simulink model "Ex3_3"  (R2019b)
settings: Solver=VariableStepAuto  StartTime=0.0  StopTime=inf  RelTol=1e-3
values from neighbouring files (symbols this model uses):
  attMtx = [L*k, 0, -L*k, 0; 0, L*k, 0, -L*k; b, -b, b, -b; 1, 1, 1, 1]    [Ex6_3_constants.m]
  b = 1.3678e-07    [Ex6_3_constants.m]
  D = diag([kD, kD, kD])    [Ex6_3_constants.m]
  g = [0, 0, -9.81]'    [Ex6_3_constants.m]
  I = diag([Ixx, Iyy, Izz])    [Ex6_3_constants.m]
  Ixx = 0.007    [Ex6_3_constants.m]
  Iyy = 0.007    [Ex6_3_constants.m]
  Izz = 0.012    [Ex6_3_constants.m]
  k = 8.54858e-06    [Ex6_3_constants.m]
  L = 0.17    [Ex6_3_constants.m]
  m = 0.716    [Ex6_3_constants.m]
  mmat = diag([m, m, m])    [Ex6_3_constants.m]
  posMtx = [0, -1, 0; 1, 0, 0]    [Ex6_3_constants.m]
undefined symbols (not defined in the file or in its folder): AA, BB, CC, DD, Omega
libraries: simulink x6, vrlib x1
settings Model: Creator=ubuntu  LastModifiedBy=ubuntu

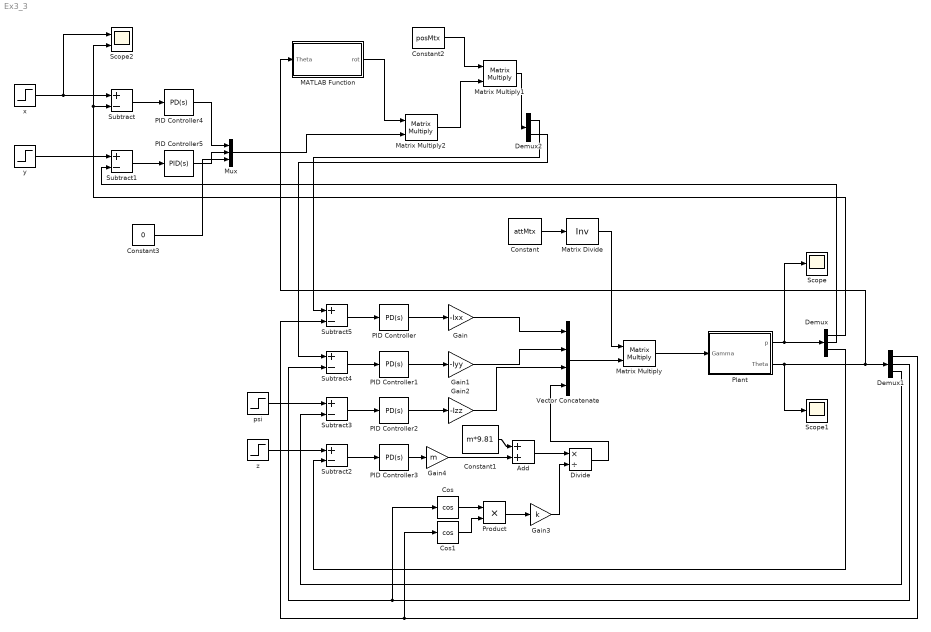
== system Ex3_3 ==
  Add : Sum
  Constant : Constant  Value=attMtx
  Constant1 : Constant  Value=m*9.81
  Constant2 : Constant  Value=posMtx
  Constant3 : Constant  Value=0
  Cos : Trigonometry  Operator=cos
  Cos1 : Trigonometry  Operator=cos
  Demux : Demux  Outputs=3
  Demux1 : Demux  Outputs=3
  Demux2 : Demux  Outputs=2
  Divide : Product  Inputs=*/
  Gain : Gain  Gain=-Ixx
  Gain1 : Gain  Gain=-Iyy
  Gain2 : Gain  Gain=-Izz
  Gain3 : Gain  Gain=k
  Gain4 : Gain  Gain=m
  MATLAB Function : MATLAB Function  TreatAsAtomicUnit=on
  Matrix Divide : Product  Inputs=/  Multiplication=Matrix(*)
  Matrix Multiply : Product  Multiplication=Matrix(*)
  Matrix Multiply1 : Product  Multiplication=Matrix(*)
  Matrix Multiply2 : Product  Multiplication=Matrix(*)
  Mux : Mux  Inputs=3
  PID Controller : simulink/Continuous/PID Controller  Controller=PD  Form=Parallel  TimeDomain=Continuous-time  SampleTime=-1  IntegratorMethod=Forward Euler  FilterMethod=Forward Euler  ControllerParametersSource=internal  P=-0.0546888957134836  I=1  D=-2.49980858398748  UseFilter=on  N=285.7069940104  TunerSelectOption=Transfer Function Based (PID Tuner App)  InitialConditionSource=internal  InitialConditionForIntegrator=0  InitialConditionForFilter=0  DifferentiatorICPrevScaledInput=0  ExternalReset=none  TrackingMode=off  Kt=1  LimitOutput=off  UpperSaturationLimit=inf  LowerSaturationLimit=-inf  LinearizeAsGain=on  AntiWindupMode=none  Kb=1  POutMin=[]  POutMax=[]  IOutMin=[]  IOutMax=[]  DOutMin=[]  DOutMax=[]  NOutMin=[]  NOutMax=[]  SumOutMin=[]  SumOutMax=[]  SaturationOutMin=[]  SaturationOutMax=[]  PParamMin=[]  PParamMax=[]  IParamMin=[]  IParamMax=[]  DParamMin=[]  DParamMax=[]  NParamMin=[]  NParamMax=[]  KbParamMin=[]  KbParamMax=[]  KtParamMin=[]  KtParamMax=[]  KbOutMin=[]  KbOutMax=[]  KtOutMin=[]  KtOutMax=[]  IntegratorOutMin=[]  IntegratorOutMax=[]  FilterOutMin=[]  FilterOutMax=[]  SumI1OutMin=[]  SumI1OutMax=[]  SumI2OutMin=[]  SumI2OutMax=[]  SumI3OutMin=[]  SumI3OutMax=[]  SumI4OutMin=[]  SumI4OutMax=[]  SumDOutMin=[]  SumDOutMax=[]  DifferentiatorOutMin=[]  DifferentiatorOutMax=[]  FilterDiffOutCoefMin=[]  FilterDiffOutCoefMax=[]  ReciprocalOutMin=[]  ReciprocalOutMax=[]  SumDenOutMin=[]  SumDenOutMax=[]  SumNumOutMin=[]  SumNumOutMax=[]  DivideOutMin=[]  DivideOutMax=[]  IntegratorContinuousStateAttributes=''  IntegratorStateMustResolveToSignalObject=off  IntegratorRTWStateStorageClass=Auto  FilterContinuousStateAttributes=''  FilterStateMustResolveToSignalObject=off  FilterRTWStateStorageClass=Auto  ParallelPVariant=InternalParameters  IdealPVariant=Disabled  IVariant=Disabled  DVariant=InternalParameters  IntegratorVariant=Disabled  SatVariant=Disabled  AWVariant=Disabled  PCopyVariant=Disabled  TRVariant=Disabled  FdbkBlocksVariant=Forward  IdealPFdbkVariant=Disabled  SatFdbkVariant=Disabled  DerivativeFilterVariant=ContFilter  NVariant=InternalParameters  NCopyVariant=Disabled  FilterICVariant=InternalICsFilter  IntegratorICVariant=Disabled  ExternalResetVariant=Disabled  TRSumVariant=Passthrough  SumFdbkVariant=Disabled  SumVariant=Sum_PD
  PID Controller1 : simulink/Continuous/PID Controller  Controller=PD  Form=Parallel  TimeDomain=Continuous-time  SampleTime=-1  IntegratorMethod=Forward Euler  FilterMethod=Forward Euler  ControllerParametersSource=internal  P=-0.0546888957134836  I=1  D=-2.49980858398748  UseFilter=on  N=285.7069940104  TunerSelectOption=Transfer Function Based (PID Tuner App)  InitialConditionSource=internal  InitialConditionForIntegrator=0  InitialConditionForFilter=0  DifferentiatorICPrevScaledInput=0  ExternalReset=none  TrackingMode=off  Kt=1  LimitOutput=off  UpperSaturationLimit=inf  LowerSaturationLimit=-inf  LinearizeAsGain=on  AntiWindupMode=none  Kb=1  POutMin=[]  POutMax=[]  IOutMin=[]  IOutMax=[]  DOutMin=[]  DOutMax=[]  NOutMin=[]  NOutMax=[]  SumOutMin=[]  SumOutMax=[]  SaturationOutMin=[]  SaturationOutMax=[]  PParamMin=[]  PParamMax=[]  IParamMin=[]  IParamMax=[]  DParamMin=[]  DParamMax=[]  NParamMin=[]  NParamMax=[]  KbParamMin=[]  KbParamMax=[]  KtParamMin=[]  KtParamMax=[]  KbOutMin=[]  KbOutMax=[]  KtOutMin=[]  KtOutMax=[]  IntegratorOutMin=[]  IntegratorOutMax=[]  FilterOutMin=[]  FilterOutMax=[]  SumI1OutMin=[]  SumI1OutMax=[]  SumI2OutMin=[]  SumI2OutMax=[]  SumI3OutMin=[]  SumI3OutMax=[]  SumI4OutMin=[]  SumI4OutMax=[]  SumDOutMin=[]  SumDOutMax=[]  DifferentiatorOutMin=[]  DifferentiatorOutMax=[]  FilterDiffOutCoefMin=[]  FilterDiffOutCoefMax=[]  ReciprocalOutMin=[]  ReciprocalOutMax=[]  SumDenOutMin=[]  SumDenOutMax=[]  SumNumOutMin=[]  SumNumOutMax=[]  DivideOutMin=[]  DivideOutMax=[]  IntegratorContinuousStateAttributes=''  IntegratorStateMustResolveToSignalObject=off  IntegratorRTWStateStorageClass=Auto  FilterContinuousStateAttributes=''  FilterStateMustResolveToSignalObject=off  FilterRTWStateStorageClass=Auto  ParallelPVariant=InternalParameters  IdealPVariant=Disabled  IVariant=Disabled  DVariant=InternalParameters  IntegratorVariant=Disabled  SatVariant=Disabled  AWVariant=Disabled  PCopyVariant=Disabled  TRVariant=Disabled  FdbkBlocksVariant=Forward  IdealPFdbkVariant=Disabled  SatFdbkVariant=Disabled  DerivativeFilterVariant=ContFilter  NVariant=InternalParameters  NCopyVariant=Disabled  FilterICVariant=InternalICsFilter  IntegratorICVariant=Disabled  ExternalResetVariant=Disabled  TRSumVariant=Passthrough  SumFdbkVariant=Disabled  SumVariant=Sum_PD
  PID Controller2 : simulink/Continuous/PID Controller  Controller=PD  Form=Parallel  TimeDomain=Continuous-time  SampleTime=-1  IntegratorMethod=Forward Euler  FilterMethod=Forward Euler  ControllerParametersSource=internal  P=-0.054688895713367  I=1  D=-2.49980858398216  UseFilter=on  N=285.7069940104  TunerSelectOption=Transfer Function Based (PID Tuner App)  InitialConditionSource=internal  InitialConditionForIntegrator=0  InitialConditionForFilter=0  DifferentiatorICPrevScaledInput=0  ExternalReset=none  TrackingMode=off  Kt=1  LimitOutput=off  UpperSaturationLimit=inf  LowerSaturationLimit=-inf  LinearizeAsGain=on  AntiWindupMode=none  Kb=1  POutMin=[]  POutMax=[]  IOutMin=[]  IOutMax=[]  DOutMin=[]  DOutMax=[]  NOutMin=[]  NOutMax=[]  SumOutMin=[]  SumOutMax=[]  SaturationOutMin=[]  SaturationOutMax=[]  PParamMin=[]  PParamMax=[]  IParamMin=[]  IParamMax=[]  DParamMin=[]  DParamMax=[]  NParamMin=[]  NParamMax=[]  KbParamMin=[]  KbParamMax=[]  KtParamMin=[]  KtParamMax=[]  KbOutMin=[]  KbOutMax=[]  KtOutMin=[]  KtOutMax=[]  IntegratorOutMin=[]  IntegratorOutMax=[]  FilterOutMin=[]  FilterOutMax=[]  SumI1OutMin=[]  SumI1OutMax=[]  SumI2OutMin=[]  SumI2OutMax=[]  SumI3OutMin=[]  SumI3OutMax=[]  SumI4OutMin=[]  SumI4OutMax=[]  SumDOutMin=[]  SumDOutMax=[]  DifferentiatorOutMin=[]  DifferentiatorOutMax=[]  FilterDiffOutCoefMin=[]  FilterDiffOutCoefMax=[]  ReciprocalOutMin=[]  ReciprocalOutMax=[]  SumDenOutMin=[]  SumDenOutMax=[]  SumNumOutMin=[]  SumNumOutMax=[]  DivideOutMin=[]  DivideOutMax=[]  IntegratorContinuousStateAttributes=''  IntegratorStateMustResolveToSignalObject=off  IntegratorRTWStateStorageClass=Auto  FilterContinuousStateAttributes=''  FilterStateMustResolveToSignalObject=off  FilterRTWStateStorageClass=Auto  ParallelPVariant=InternalParameters  IdealPVariant=Disabled  IVariant=Disabled  DVariant=InternalParameters  IntegratorVariant=Disabled  SatVariant=Disabled  AWVariant=Disabled  PCopyVariant=Disabled  TRVariant=Disabled  FdbkBlocksVariant=Forward  IdealPFdbkVariant=Disabled  SatFdbkVariant=Disabled  DerivativeFilterVariant=ContFilter  NVariant=InternalParameters  NCopyVariant=Disabled  FilterICVariant=InternalICsFilter  IntegratorICVariant=Disabled  ExternalResetVariant=Disabled  TRSumVariant=Passthrough  SumFdbkVariant=Disabled  SumVariant=Sum_PD
  PID Controller3 : simulink/Continuous/PID Controller  Controller=PD  Form=Parallel  TimeDomain=Continuous-time  SampleTime=-1  IntegratorMethod=Forward Euler  FilterMethod=Forward Euler  ControllerParametersSource=internal  P=0.00875107669312752  I=0.000153136025532483  D=1.00002095266386  UseFilter=on  N=114.28279760416  TunerSelectOption=Transfer Function Based (PID Tuner App)  InitialConditionSource=internal  InitialConditionForIntegrator=0  InitialConditionForFilter=0  DifferentiatorICPrevScaledInput=0  ExternalReset=none  TrackingMode=off  Kt=1  LimitOutput=off  UpperSaturationLimit=inf  LowerSaturationLimit=-inf  LinearizeAsGain=on  AntiWindupMode=none  Kb=1  POutMin=[]  POutMax=[]  IOutMin=[]  IOutMax=[]  DOutMin=[]  DOutMax=[]  NOutMin=[]  NOutMax=[]  SumOutMin=[]  SumOutMax=[]  SaturationOutMin=[]  SaturationOutMax=[]  PParamMin=[]  PParamMax=[]  IParamMin=[]  IParamMax=[]  DParamMin=[]  DParamMax=[]  NParamMin=[]  NParamMax=[]  KbParamMin=[]  KbParamMax=[]  KtParamMin=[]  KtParamMax=[]  KbOutMin=[]  KbOutMax=[]  KtOutMin=[]  KtOutMax=[]  IntegratorOutMin=[]  IntegratorOutMax=[]  FilterOutMin=[]  FilterOutMax=[]  SumI1OutMin=[]  SumI1OutMax=[]  SumI2OutMin=[]  SumI2OutMax=[]  SumI3OutMin=[]  SumI3OutMax=[]  SumI4OutMin=[]  SumI4OutMax=[]  SumDOutMin=[]  SumDOutMax=[]  DifferentiatorOutMin=[]  DifferentiatorOutMax=[]  FilterDiffOutCoefMin=[]  FilterDiffOutCoefMax=[]  ReciprocalOutMin=[]  ReciprocalOutMax=[]  SumDenOutMin=[]  SumDenOutMax=[]  SumNumOutMin=[]  SumNumOutMax=[]  DivideOutMin=[]  DivideOutMax=[]  IntegratorContinuousStateAttributes=''  IntegratorStateMustResolveToSignalObject=off  IntegratorRTWStateStorageClass=Auto  FilterContinuousStateAttributes=''  FilterStateMustResolveToSignalObject=off  FilterRTWStateStorageClass=Auto  ParallelPVariant=InternalParameters  IdealPVariant=Disabled  IVariant=Disabled  DVariant=InternalParameters  IntegratorVariant=Disabled  SatVariant=Disabled  AWVariant=Disabled  PCopyVariant=Disabled  TRVariant=Disabled  FdbkBlocksVariant=Forward  IdealPFdbkVariant=Disabled  SatFdbkVariant=Disabled  DerivativeFilterVariant=ContFilter  NVariant=InternalParameters  NCopyVariant=Disabled  FilterICVariant=InternalICsFilter  IntegratorICVariant=Disabled  ExternalResetVariant=Disabled  TRSumVariant=Passthrough  SumFdbkVariant=Disabled  SumVariant=Sum_PD
  PID Controller4 : simulink/Continuous/PID Controller  Controller=PD  Form=Parallel  TimeDomain=Continuous-time  SampleTime=-1  IntegratorMethod=Forward Euler  FilterMethod=Forward Euler  ControllerParametersSource=internal  P=-0.000952303322901341  I=1  D=-0.108823555042164  UseFilter=on  N=114.28279760416  TunerSelectOption=Transfer Function Based (PID Tuner App)  InitialConditionSource=internal  InitialConditionForIntegrator=0  InitialConditionForFilter=0  DifferentiatorICPrevScaledInput=0  ExternalReset=none  TrackingMode=off  Kt=1  LimitOutput=off  UpperSaturationLimit=inf  LowerSaturationLimit=-inf  LinearizeAsGain=on  AntiWindupMode=none  Kb=1  POutMin=[]  POutMax=[]  IOutMin=[]  IOutMax=[]  DOutMin=[]  DOutMax=[]  NOutMin=[]  NOutMax=[]  SumOutMin=[]  SumOutMax=[]  SaturationOutMin=[]  SaturationOutMax=[]  PParamMin=[]  PParamMax=[]  IParamMin=[]  IParamMax=[]  DParamMin=[]  DParamMax=[]  NParamMin=[]  NParamMax=[]  KbParamMin=[]  KbParamMax=[]  KtParamMin=[]  KtParamMax=[]  KbOutMin=[]  KbOutMax=[]  KtOutMin=[]  KtOutMax=[]  IntegratorOutMin=[]  IntegratorOutMax=[]  FilterOutMin=[]  FilterOutMax=[]  SumI1OutMin=[]  SumI1OutMax=[]  SumI2OutMin=[]  SumI2OutMax=[]  SumI3OutMin=[]  SumI3OutMax=[]  SumI4OutMin=[]  SumI4OutMax=[]  SumDOutMin=[]  SumDOutMax=[]  DifferentiatorOutMin=[]  DifferentiatorOutMax=[]  FilterDiffOutCoefMin=[]  FilterDiffOutCoefMax=[]  ReciprocalOutMin=[]  ReciprocalOutMax=[]  SumDenOutMin=[]  SumDenOutMax=[]  SumNumOutMin=[]  SumNumOutMax=[]  DivideOutMin=[]  DivideOutMax=[]  IntegratorContinuousStateAttributes=''  IntegratorStateMustResolveToSignalObject=off  IntegratorRTWStateStorageClass=Auto  FilterContinuousStateAttributes=''  FilterStateMustResolveToSignalObject=off  FilterRTWStateStorageClass=Auto  ParallelPVariant=InternalParameters  IdealPVariant=Disabled  IVariant=Disabled  DVariant=InternalParameters  IntegratorVariant=Disabled  SatVariant=Disabled  AWVariant=Disabled  PCopyVariant=Disabled  TRVariant=Disabled  FdbkBlocksVariant=Forward  IdealPFdbkVariant=Disabled  SatFdbkVariant=Disabled  DerivativeFilterVariant=ContFilter  NVariant=InternalParameters  NCopyVariant=Disabled  FilterICVariant=InternalICsFilter  IntegratorICVariant=Disabled  ExternalResetVariant=Disabled  TRSumVariant=Passthrough  SumFdbkVariant=Disabled  SumVariant=Sum_PD
  PID Controller5 : simulink/Continuous/PID Controller  Controller=PID  Form=Parallel  TimeDomain=Continuous-time  SampleTime=-1  IntegratorMethod=Forward Euler  FilterMethod=Forward Euler  ControllerParametersSource=internal  P=1  I=1  D=0  UseFilter=on  N=100  TunerSelectOption=Transfer Function Based (PID Tuner App)  InitialConditionSource=internal  InitialConditionForIntegrator=0  InitialConditionForFilter=0  DifferentiatorICPrevScaledInput=0  ExternalReset=none  TrackingMode=off  Kt=1  LimitOutput=off  UpperSaturationLimit=inf  LowerSaturationLimit=-inf  LinearizeAsGain=on  AntiWindupMode=none  Kb=1  POutMin=[]  POutMax=[]  IOutMin=[]  IOutMax=[]  DOutMin=[]  DOutMax=[]  NOutMin=[]  NOutMax=[]  SumOutMin=[]  SumOutMax=[]  SaturationOutMin=[]  SaturationOutMax=[]  PParamMin=[]  PParamMax=[]  IParamMin=[]  IParamMax=[]  DParamMin=[]  DParamMax=[]  NParamMin=[]  NParamMax=[]  KbParamMin=[]  KbParamMax=[]  KtParamMin=[]  KtParamMax=[]  KbOutMin=[]  KbOutMax=[]  KtOutMin=[]  KtOutMax=[]  IntegratorOutMin=[]  IntegratorOutMax=[]  FilterOutMin=[]  FilterOutMax=[]  SumI1OutMin=[]  SumI1OutMax=[]  SumI2OutMin=[]  SumI2OutMax=[]  SumI3OutMin=[]  SumI3OutMax=[]  SumI4OutMin=[]  SumI4OutMax=[]  SumDOutMin=[]  SumDOutMax=[]  DifferentiatorOutMin=[]  DifferentiatorOutMax=[]  FilterDiffOutCoefMin=[]  FilterDiffOutCoefMax=[]  ReciprocalOutMin=[]  ReciprocalOutMax=[]  SumDenOutMin=[]  SumDenOutMax=[]  SumNumOutMin=[]  SumNumOutMax=[]  DivideOutMin=[]  DivideOutMax=[]  IntegratorContinuousStateAttributes=''  IntegratorStateMustResolveToSignalObject=off  IntegratorRTWStateStorageClass=Auto  FilterContinuousStateAttributes=''  FilterStateMustResolveToSignalObject=off  FilterRTWStateStorageClass=Auto  ParallelPVariant=InternalParameters  IdealPVariant=Disabled  IVariant=InternalParameters  DVariant=InternalParameters  IntegratorVariant=Continuous  SatVariant=Disabled  AWVariant=Passthrough  PCopyVariant=Disabled  TRVariant=Disabled  FdbkBlocksVariant=Forward  IdealPFdbkVariant=Disabled  SatFdbkVariant=Disabled  DerivativeFilterVariant=ContFilter  NVariant=InternalParameters  NCopyVariant=Disabled  FilterICVariant=InternalICsFilter  IntegratorICVariant=InternalICs  ExternalResetVariant=Disabled  TRSumVariant=Passthrough  SumFdbkVariant=Disabled  SumVariant=Sum_PID
  Plant : Subsystem
  Product : Product
  Scope : Scope
  Scope1 : Scope
  Scope2 : Scope  NumInputPorts=2
  Subtract{,1..5} (6 alike) : Sum  Inputs=+-
  Vector Concatenate : Concatenate  NumInputs=4
  psi : Step  After=0  SampleTime=0
  "x " : Step  After=10  SampleTime=0
  "y " : Step  After=0  SampleTime=0
  z : Step  After=0  SampleTime=0
  wires:
  Plant/2("Theta ") -> Scope1/1, MATLAB Function/1(Theta), Demux1/1
  Gain1/1 -> Vector Concatenate/2
  Demux/3 -> Subtract2/2
  Matrix Multiply/1 -> Plant/1(Gamma)
  PID Controller/1 -> Gain/1
  Demux1/1 -> Cos1/1, Subtract5/2
  Subtract4/1 -> PID Controller1/1
  Matrix Divide/1 -> Matrix Multiply/1
  Cos/1 -> Product/1
  Cos1/1 -> Product/2
  PID Controller1/1 -> Gain1/1
  Add/1 -> Divide/1
  Demux1/2 -> Cos/1, Subtract4/2
  Subtract3/1 -> PID Controller2/1
  Plant/1(p) -> Scope/1, Demux/1
  psi/1 -> Subtract3/1
  Subtract2/1 -> PID Controller3/1
  Vector Concatenate/1 -> Matrix Multiply/2
  z/1 -> Subtract2/1
  Constant1/1 -> Add/1
  PID Controller2/1 -> Gain2/1
  PID Controller3/1 -> Gain4/1
  Product/1 -> Gain3/1
  Gain2/1 -> Vector Concatenate/3
  Demux1/3 -> Subtract3/2
  Gain3/1 -> Divide/2
  Gain4/1 -> Add/2
  Gain/1 -> Vector Concatenate/1
  Divide/1 -> Vector Concatenate/4
  Constant/1 -> Matrix Divide/1
  Subtract5/1 -> PID Controller/1
  Subtract/1 -> PID Controller4/1
  Subtract1/1 -> PID Controller5/1
  PID Controller4/1 -> Mux/1
  PID Controller5/1 -> Mux/2
  Mux/1 -> Matrix Multiply2/2
  "x "/1 -> Scope2/1, Subtract/1
  "y "/1 -> Subtract1/1
  Demux/1 -> Scope2/2, Subtract/2
  Demux/2 -> Subtract1/2
  Demux2/2 -> Subtract4/1
  Demux2/1 -> Subtract5/1
  Constant3/1 -> Mux/3
  Constant2/1 -> Matrix Multiply1/1
  MATLAB Function/1(rot) -> Matrix Multiply2/1
  Matrix Multiply2/1 -> Matrix Multiply1/2
  Matrix Multiply1/1 -> Demux2/1

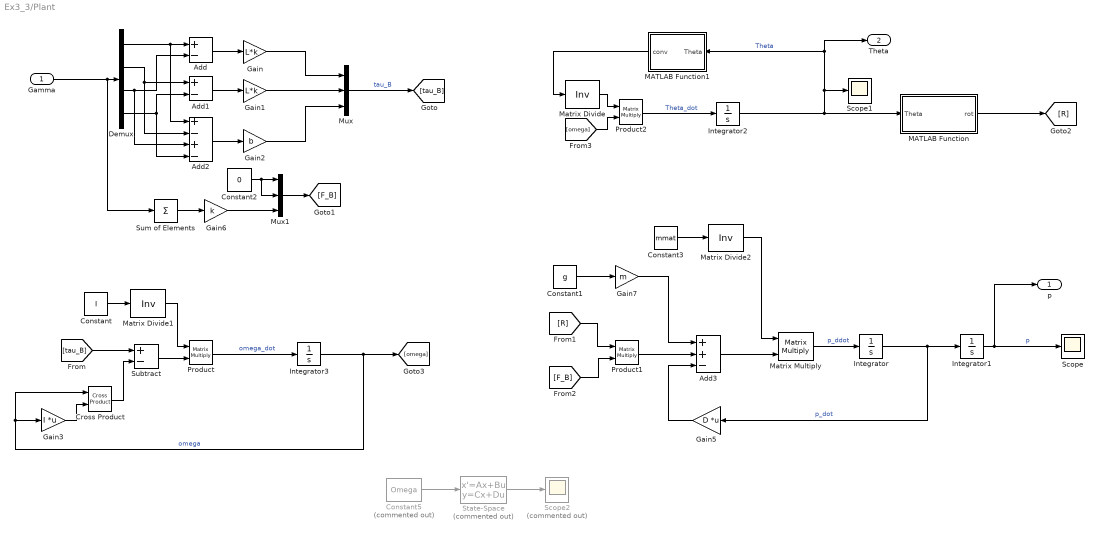
== system Ex3_3/Plant ==
  Gamma : Inport
  Add : Sum  Inputs=+-
  Add1 : Sum  Inputs=+-
  Add2 : Sum  Inputs=+-+-
  Add3 : Sum  Inputs=++-
  Constant : Constant  Value=I
  Constant1 : Constant  Value=g
  Constant2 : Constant  Value=0
  Constant3 : Constant  Value=mmat
  Constant5 : Constant  Commented=on  Value=Omega
  Cross Product : vrlib/Utilities/Cross Product
      settings: SourceProductName=Simulink
  Demux : Demux
  Gain : Gain  Gain=L*k
  Gain1 : Gain  Gain=L*k
  Gain2 : Gain  Gain=b
  Gain3 : Gain  Gain=I  Multiplication=Matrix(K*u)
  Gain5 : Gain  Gain=D  Multiplication=Matrix(K*u)
  Gain6 : Gain  Gain=k
  Gain7 : Gain  Gain=m
  Integrator : Integrator  InitialCondition=[0, 0, 0]'  ContinuousStateAttributes='p_dot'
  Integrator1 : Integrator  InitialCondition=[0, 0, 0]'  ContinuousStateAttributes='p'
  Integrator2 : Integrator  InitialCondition=[0, 0, 0]'  ContinuousStateAttributes='orientation'
  Integrator3 : Integrator  InitialCondition=[0, 0, 0]'  ContinuousStateAttributes='omega'
  MATLAB Function : MATLAB Function  TreatAsAtomicUnit=on
  MATLAB Function1 : MATLAB Function  TreatAsAtomicUnit=on
  Matrix Divide : Product  Inputs=/  Multiplication=Matrix(*)
  Matrix Divide1 : Product  Inputs=/  Multiplication=Matrix(*)
  Matrix Divide2 : Product  Inputs=/  Multiplication=Matrix(*)
  Matrix Multiply : Product  Multiplication=Matrix(*)
  Mux : Mux  Inputs=3
  Mux1 : Mux  Inputs=3
  Product : Product  Multiplication=Matrix(*)
  Product1 : Product  Multiplication=Matrix(*)
  Product2 : Product  Multiplication=Matrix(*)
  Scope : Scope
  Scope1 : Scope
  Scope2 : Scope  Commented=on
  State-Space : StateSpace  Commented=on  A=AA  B=BB  C=CC  D=DD  InitialCondition=[0,0,0,0,0,0,0,0,0,0,0,0]
  Subtract : Sum  Inputs=+-
  Sum of Elements : Sum  Inputs=+
  p : Outport
  "Theta " : Outport  Port=2
  wires:
  Add2/1 -> Gain2/1
  Constant5/1 -> State-Space/1
  Gain2/1 -> Mux/3
  Constant1/1 -> Gain7/1
  Gamma/1 -> Sum of Elements/1, Demux/1
  Constant2/1 -> Mux1/1, Mux1/2
  Add1/1 -> Gain1/1
  Gain/1 -> Mux/1
  [tau_B] -> Subtract/1
  Add/1 -> Gain/1
  MATLAB Function1/1(conv) -> Matrix Divide/1
  Demux/2 -> Add2/2, Add1/1
  MATLAB Function/1(rot) -> [R]
  Matrix Divide2/1 -> Matrix Multiply/1
  Demux/3 -> Add2/3, Add/2
  State-Space/1 -> Scope2/1
  [omega] -> Product2/2
  Integrator/1 -> Gain5/1, Integrator1/1  "p_dot"
  Matrix Multiply/1 -> Integrator/1  "p_ddot"
  [R] -> Product1/1
  Mux1/1 -> [F_B]
  Product1/1 -> Add3/2
  Constant3/1 -> Matrix Divide2/1
  Product/1 -> Integrator3/1  "omega_dot"
  Cross Product/1 -> Subtract/2
  Constant/1 -> Matrix Divide1/1
  Product2/1 -> Integrator2/1  "Theta_dot"
  Matrix Divide1/1 -> Product/1
  [F_B] -> Product1/2
  Demux/1 -> Add2/1, Add/1
  Subtract/1 -> Product/2
  Gain7/1 -> Add3/1
  Integrator3/1 -> [omega], Gain3/1, Cross Product/1  "omega"
  Gain5/1 -> Add3/3
  Gain1/1 -> Mux/2
  Mux/1 -> [tau_B]  "tau_B"
  Gain3/1 -> Cross Product/2
  Add3/1 -> Matrix Multiply/2
  Matrix Divide/1 -> Product2/1
  Integrator2/1 -> "Theta "/1, MATLAB Function1/1(Theta), Scope1/1, MATLAB Function/1(Theta)  "Theta"
  Gain6/1 -> Mux1/3
  Demux/4 -> Add1/2, Add2/4
  Integrator1/1 -> p/1, Scope/1  "p"
  Sum of Elements/1 -> Gain6/1

== matlab function Ex3_3/Plant/MATLAB Function1 ==
  data: Theta input; conv output
function conv = ConvMtx(Theta)

the = Theta(2);
phi = Theta(1);

conv = [1, 0, -sin(the); 0, cos(phi), cos(the)*sin(phi); 0, -sin(phi), cos(the)*cos(phi)];

== matlab function Ex3_3/Plant/MATLAB Function ==
  data: Theta input; rot output
function rot = RotMtx(Theta)

phi = Theta(1);
the = Theta(2);
psi = Theta(3);

rot = [
    cos(psi)*cos(the), cos(psi)*sin(the)*sin(phi)-sin(psi)*cos(phi), cos(psi)*sin(the)*cos(phi)+sin(psi)*sin(phi);
    sin(psi)*cos(the), sin(psi)*sin(the)*sin(phi)+cos(psi)*cos(phi), sin(psi)*sin(the)*cos(phi)-cos(psi)*sin(phi);
    -sin(the), cos(the)*sin(phi), cos(the)*cos(phi)
    ]';

== matlab function Ex3_3/MATLAB Function ==
  data: Theta input; rot output
function rot = RotMtx(Theta)

phi = Theta(1);
the = Theta(2);
psi = Theta(3);

rot = [
    cos(psi)*cos(the), cos(psi)*sin(the)*sin(phi)-sin(psi)*cos(phi), cos(psi)*sin(the)*cos(phi)+sin(psi)*sin(phi);
    sin(psi)*cos(the), sin(psi)*sin(the)*sin(phi)+cos(psi)*cos(phi), sin(psi)*sin(the)*cos(phi)-cos(psi)*sin(phi);
    -sin(the), cos(the)*sin(phi), cos(the)*cos(phi)
    ]';
